simulink model "sea_tuning"  (R2014b)
settings: Solver=FixedStepDiscrete  StartTime=0.0  StopTime=inf  FixedStep=sample_time  RelTol=1e-3
undefined symbols (not defined in the file): A1_notch_f1, A2_notch_f1, B1_notch_f1, B2_notch_f1, back_left_triangle_period, back_left_triangle_wave_midpoint, back_left_triangle_wave_speed, back_right_triangle_period, back_right_triangle_wave_midpoint, back_right_triangle_wave_speed, boom_mount_angle, commanded_spring_torque, control_start_time, enable_left_step, enable_right_step, front_left_triangle_period, front_left_triangle_wave_midpoint, front_left_triangle_wave_speed, front_right_triangle_period, front_right_triangle_wave_midpoint, front_right_triangle_wave_speed, g, K_notch_f1, k_sea, kd_lateral, kd_sea_tuning, kd_swing_trajectory, kp_lateral, kp_sea_tuning, kp_swing_trajectory, l_seg, lateral_offset, lowest_commanded_spring_torque, m_leg_motor, max_sagittal_desired_swing_torque, max_sagittal_loaded_torque, max_sagittal_unloaded_torque, max_torque_lateral, maximum_lateral_angle, minimum_lateral_angle, sample_time, sea_coulomb_friction_direction_switch_sensitivity_tuning, sea_coulomb_friction_tuning, spring_torque_step_period
libraries: simulink x3
settings Model: xpc_rtwmakecfg_data=_xpcethercatlib_  BufferReuse=off  Creator=wmartin  LastModifiedBy=wmartin
settings SolverCC: EnableConcurrentExecution=on
settings DataIOCC: MaxDataPoints=1000000000  SaveFormat=StructureWithTime
settings OptimizationCC: BlockReduction=off  OptimizeBlockIOStorage=off  BufferReuse=off  GlobalBufferReuse=off  ExpressionFolding=off  ExpressionDepthLimit=2147483647  LocalBlockOutputs=off  SimCompilerOptimization=On
settings DebuggingCC: UnderspecifiedInitializationDetection=Classic  MergeDetectMultiDrivingBlocksExec=none  StateNameClashWarn=warning
settings HardwareCC: ProdIntDivRoundTo=Zero  ProdEndianess=LittleEndian  ProdLongLongMode=on  ProdHWDeviceType=Generic->32-bit x86 compatible
settings ModelReferenceCC: UpdateModelReferenceTargets=IfOutOfDate  EnableParallelModelReferenceBuilds=on
settings RTWCC: SystemTargetFile=slrt.tlc  TemplateMakefile=slrt_default_tmf  Description=Simulink Real-Time  RTWVerbose=off  ProcessScript=slrt_make_rtw_hook  RTWCompilerOptimization=On
settings CodeAppCC: MaxIdLength=256
settings SimulinkRealTimeCC: GeneratePreprocessorConditionals=Disable all  EnableShiftOperators=on  RL32LogBufSizeModifier=100000000

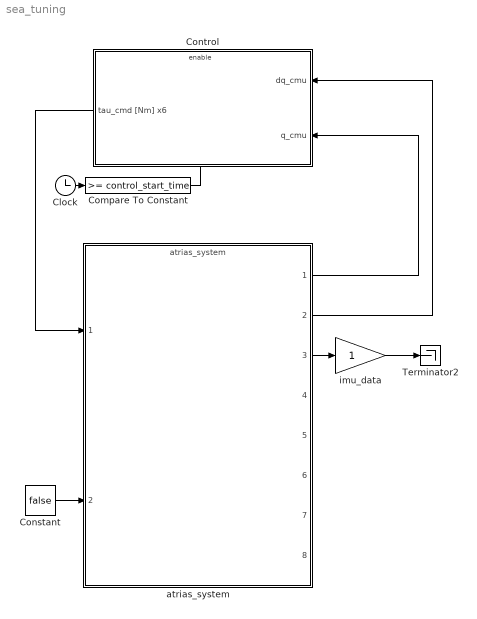
== system sea_tuning ==
  Clock : Clock
  Compare To Constant : simulink/Logic and Bit Operations/Compare To Constant  relop=>=  const=control_start_time  OutDataTypeStr=boolean
  Constant : Constant  Value=false
  Control : Subsystem
  Terminator2 : Terminator
  atrias_system : ModelReference  ModelNameDialog=atrias_system  SimulationMode=Normal  ModelReferenceVersion=1.2647  CopyOfModelName=atrias_system  DefaultDataLogging=on
  imu_data : Gain
  wires:
  Clock/1 -> Compare To Constant/1
  Compare To Constant/1 -> Control/Enable
  atrias_system/1 -> Control/2(q_cmu)
  atrias_system/2 -> Control/1(dq_cmu)
  Constant/1 -> atrias_system/2
  Control/1(tau_cmd [Nm] x6) -> atrias_system/1
  imu_data/1 -> Terminator2/1
  atrias_system/3 -> imu_data/1

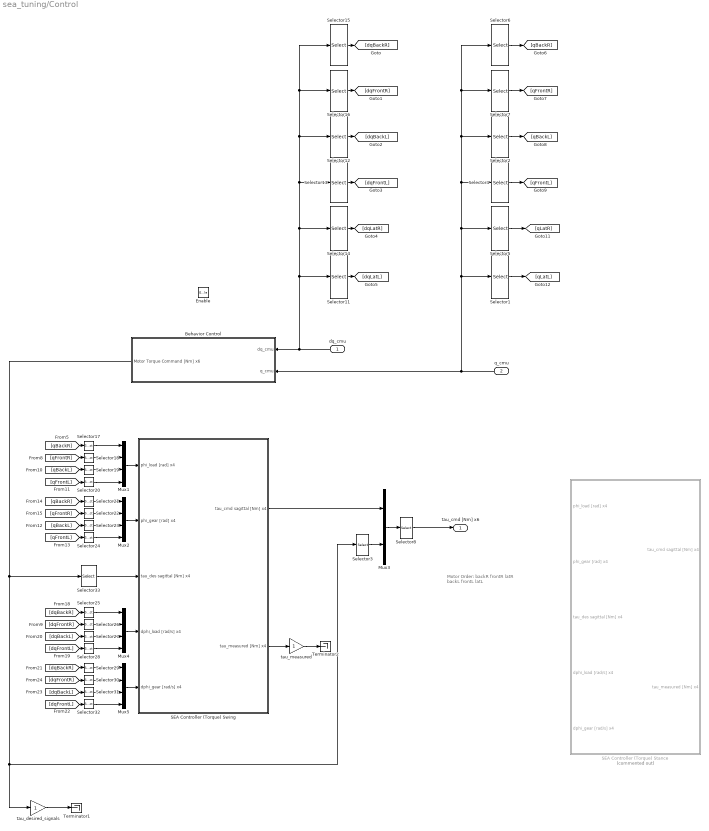
== system sea_tuning/Control ==
  note: Motor Order:
      |
      | backR
      | frontR
      | latR
      | backL
      | frontL
      | latL
  dq_cmu : Inport
  q_cmu : Inport  Port=2
  Enable : EnablePort  StatesWhenEnabling=reset
  Behavior Control : Subsystem
  Mux{1..2,4..5} (4 alike) : Mux
  Mux3 : Mux  Inputs=2
  SEA Controller (Torque) Stance : Subsystem  Commented=on
  SEA Controller (Torque) Swing : Subsystem
  Selector1 : Selector  InputPortWidth=13  Indices=[10]
  Selector11 : Selector  InputPortWidth=13  Indices=[10]
  Selector12 : Selector  InputPortWidth=13  Indices=[5 6]
  Selector13 : Selector  InputPortWidth=13  Indices=[7 8]
  Selector14 : Selector  InputPortWidth=13  Indices=[9]
  Selector15 : Selector  InputPortWidth=13  Indices=[1 2]
  Selector16 : Selector  InputPortWidth=13  Indices=[3 4]
  Selector{17..20,25..28} (8 alike) : Selector  InputPortWidth=2  Indices=[1]
  Selector2 : Selector  InputPortWidth=13  Indices=[5 6]
  Selector{21..24,29..32} (8 alike) : Selector  InputPortWidth=2  Indices=[2]
  Selector3 : Selector  InputPortWidth=6  Indices=[3 6]
  Selector33 : Selector  InputPortWidth=6  Indices=[1 2 4 5]
  Selector4 : Selector  InputPortWidth=13  Indices=[7 8]
  Selector5 : Selector  InputPortWidth=13  Indices=[9]
  Selector6 : Selector  InputPortWidth=13  Indices=[1 2]
  Selector7 : Selector  InputPortWidth=13  Indices=[3 4]
  Selector8 : Selector  InputPortWidth=6  Indices=[1 2 5 3 4 6]
  Terminator1 : Terminator
  Terminator2 : Terminator
  tau_desired_signals : Gain  Description=xPCTag(1)=tau_cmd_signal;
  tau_measured : Gain  Description=xPCTag(1)=tau_cmd_signal;
  tau_cmd [Nm] x6 : Outport  InitialOutput=[0 0 0 0 0 0]
  wires:
  SEA Controller (Torque) Swing/1(tau_cmd sagittal [Nm] x4) -> Mux3/1
  Behavior Control/1(Motor Torque Command [Nm] x6) -> tau_desired_signals/1, Selector3/1, Selector33/1
  Selector8/1 -> tau_cmd [Nm] x6/1
  tau_desired_signals/1 -> Terminator1/1
  Selector5/1 -> [qLatR]
  Selector1/1 -> [qLatL]
  Selector6/1 -> [qBackR]
  Selector7/1 -> [qFrontR]
  Selector2/1 -> [qBackL]
  Selector4/1 -> [qFrontL]
  q_cmu/1 -> Behavior Control/2(q_cmu), Selector2/1, Selector7/1, Selector6/1, Selector4/1, Selector5/1, Selector1/1
  dq_cmu/1 -> Selector15/1, Selector16/1, Selector12/1, Selector13/1, Selector14/1, Selector11/1, Behavior Control/1(dq_cmu)
  Selector14/1 -> [dqLatR]
  Selector11/1 -> [dqLatL]
  Selector15/1 -> [dqBackR]
  Selector16/1 -> [dqFrontR]
  Selector12/1 -> [dqBackL]
  Selector13/1 -> [dqFrontL]
  Mux1/1 -> SEA Controller (Torque) Swing/1(phi_load [rad] x4)
  [qBackR] -> Selector17/1
  Selector17/1 -> Mux1/1
  Selector19/1 -> Mux1/3
  Selector18/1 -> Mux1/2
  Selector20/1 -> Mux1/4
  [qFrontR] -> Selector18/1
  [qBackL] -> Selector19/1
  [qFrontL] -> Selector20/1
  Mux2/1 -> SEA Controller (Torque) Swing/2(phi_gear [rad] x4)
  [qBackR] -> Selector21/1
  Selector21/1 -> Mux2/1
  Selector23/1 -> Mux2/3
  Selector22/1 -> Mux2/2
  Selector24/1 -> Mux2/4
  [qFrontR] -> Selector22/1
  [qBackL] -> Selector23/1
  [qFrontL] -> Selector24/1
  Mux4/1 -> SEA Controller (Torque) Swing/4(dphi_load [rad/s] x4)
  [dqBackR] -> Selector25/1
  Selector25/1 -> Mux4/1
  Selector27/1 -> Mux4/3
  Selector26/1 -> Mux4/2
  Selector28/1 -> Mux4/4
  [dqFrontR] -> Selector26/1
  [dqBackL] -> Selector27/1
  [dqFrontL] -> Selector28/1
  Mux5/1 -> SEA Controller (Torque) Swing/5(dphi_gear [rad/s] x4)
  [dqBackR] -> Selector29/1
  Selector29/1 -> Mux5/1
  Selector31/1 -> Mux5/3
  Selector30/1 -> Mux5/2
  Selector32/1 -> Mux5/4
  [dqFrontR] -> Selector30/1
  [dqBackL] -> Selector31/1
  [dqFrontL] -> Selector32/1
  Selector33/1 -> SEA Controller (Torque) Swing/3(tau_des sagittal [Nm] x4)
  Selector3/1 -> Mux3/2
  Mux3/1 -> Selector8/1
  SEA Controller (Torque) Swing/2(tau_measured [Nm] x4) -> tau_measured/1
  tau_measured/1 -> Terminator2/1

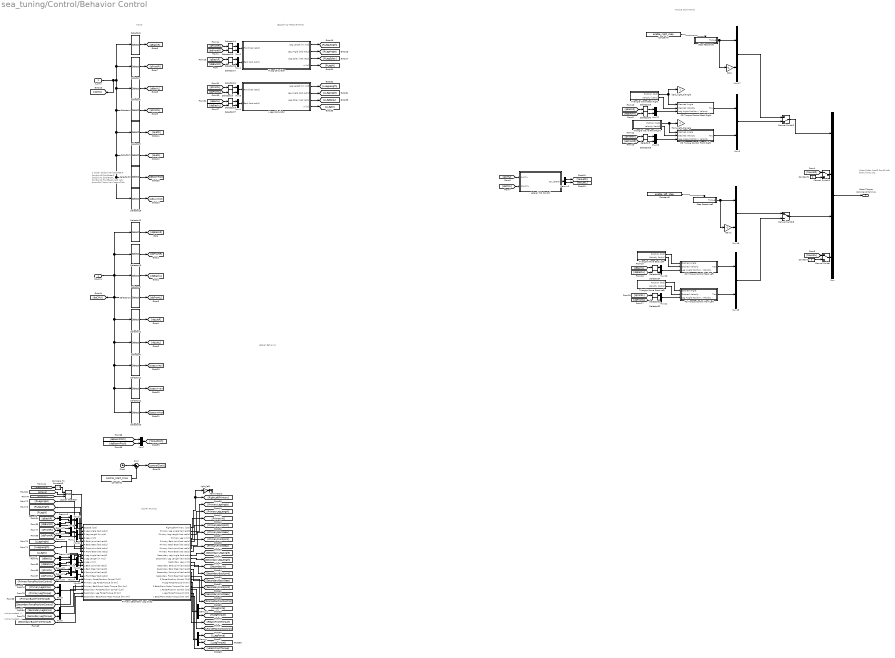
== system sea_tuning/Control/Behavior Control ==
  note: not connected -->
  note: Signal Routing
  note: Leg/Spring Measurements
  note: Lateral Behavior
  note: Torque Commands
  note: Inputs
  note: q Order:
      |
      | backJointR
      | backGearR
      | frontJointR
      | frontGearR
      |
      | backJointL
      | backGearL
      | frontJointL
      | frontGearL
      |
      | latR
      | latL
      |
      | boomRoll
      | boomYaw
      | boomPitch
  note: Motor Order:
      |
      | backR
      | frontR
      | latR
      | backL
      | frontL
      | latL
  note: not connected -->
  dq_cmu : Inport
  q_cmu : Inport  Port=2
  Clock : Clock
  Compare To Constant5 : simulink/Logic and Bit Operations/Compare To Constant  relop=>  const=2  OutDataTypeStr=boolean
  Constant : Constant  Value=0
  Constant1 : Constant  Value=0
  Constant2 : Constant  Value=control_start_time
  Constant4 : Constant  Value=enable_right_step
  Constant5 : Constant  Value=enable_left_step
  Demux{,1..10} (11 alike) : Demux  Outputs=2
  Gain : Gain  Gain=-1
  Gain1 : Gain  Gain=-1
  L Leg Calculator : Subsystem
  Lateral PID Control : Subsystem
  Logical Operator : Logic  Inputs=3  IconShape=distinctive  AllPortsSameDT=off  OutDataTypeStr=boolean
  Manual Switch : ManualSwitch
  Manual Switch1 : ManualSwitch
  Manual Switch2 : ManualSwitch  CurrentSetting=0
  Manual Switch3 : ManualSwitch
  Mux : Mux
  Mux{1..23} (23 alike) : Mux  Inputs=2
  PD Torque Control Back Left : Subsystem
  PD Torque Control Back Right : Subsystem
  PD Torque Control Front Left : Subsystem
  PD Torque Control Front Right : Subsystem
  Primary Secondary Leg Swap : Subsystem
  R Leg Calculator : Subsystem
  Selector1 : Selector  InputPortWidth=13  Indices=[10]
  Selector10 : Selector  InputPortWidth=13  Indices=[7 8]
  Selector11 : Selector  InputPortWidth=13  Indices=[9]
  Selector12 : Selector  InputPortWidth=13  Indices=[1 2]
  Selector13 : Selector  InputPortWidth=13  Indices=[3 4]
  Selector{3,14..17,24..34} (16 alike) : Selector  InputPortWidth=2  Indices=[1]
  Selector18 : Selector  InputPortWidth=13  Indices=[13]
  Selector2 : Selector  InputPortWidth=13  Indices=[5 6]
  Selector20 : Selector  InputPortWidth=13  Indices=[13]
  Selector21 : Selector  InputPortWidth=13  Indices=[11]
  Selector22 : Selector  InputPortWidth=13  Indices=[12]
  Selector23 : Selector  InputPortWidth=13  Indices=[11]
  Selector4 : Selector  InputPortWidth=13  Indices=[7 8]
  Selector5 : Selector  InputPortWidth=13  Indices=[9]
  Selector6 : Selector  InputPortWidth=13  Indices=[1 2]
  Selector7 : Selector  InputPortWidth=13  Indices=[3 4]
  Selector8 : Selector  InputPortWidth=13  Indices=[10]
  Selector9 : Selector  InputPortWidth=13  Indices=[5 6]
  Step Response : Subsystem
  Step Response2 : Subsystem
  Sum : Sum  Inputs=|+-
  Terminator2 : Terminator
  Triangle Wave Back Left : Subsystem
  Triangle Wave Back Right : Subsystem
  Triangle Wave Front Left : Subsystem
  Triangle Wave Front Right : Subsystem
  back_right_triangle : Gain
  front_right_triangle : Gain
  right_left : Gain
  Motor Torque Command [Nm] x6 : Outport  OutputWhenDisabled=reset  InitialOutput=[0 0 0 0 0 0]
  wires:
  [escape] -> Logical Operator/2
  Mux18/1 -> Manual Switch3/1
  Step Response2/1(Torque) -> Gain1/1, Mux18/1
  Step Response/1(Torque) -> Gain/1, Mux17/1
  Manual Switch/1 -> Mux/4
  Manual Switch1/1 -> Mux/2
  Mux17/1 -> Manual Switch2/1
  Primary Secondary Leg Swap/1(Right/Left Primary [1/0]) -> [RightLeftPrimary], right_left/1
  Logical Operator/1 -> Primary Secondary Leg Swap/1(escape [1/0])
  Primary Secondary Leg Swap/21(L Back/Front Motor Torque [Nm Nm]) -> [LBackFrontTorque]
  Primary Secondary Leg Swap/18(R Back/Front Motor Torque [Nm Nm]) -> [RBackFrontTorque]
  Primary Secondary Leg Swap/16(R Force/Position Control [1/0]) -> [RForcePositionControl]
  Primary Secondary Leg Swap/19(L Force/Position Control [1/0]) -> [LForcePositionControl]
  Primary Secondary Leg Swap/11(Secondary Leg w [m]) -> [SecondaryW]
  Primary Secondary Leg Swap/15(Secondary Front Gear [rad rad/s]) -> [SecondaryFrontGear]
  Primary Secondary Leg Swap/14(Secondary Front Joint [rad rad/s]) -> [SecondaryFrontJoint]
  Primary Secondary Leg Swap/13(Secondary Back Gear [rad rad/s]) -> [SecondaryBackGear]
  Primary Secondary Leg Swap/12(Secondary Back Joint [rad rad/s]) -> [SecondaryBackJoint]
  Primary Secondary Leg Swap/8(Primary Front Gear [rad rad/s]) -> [PrimaryFrontGear]
  Primary Secondary Leg Swap/7(Primary Front Joint [rad rad/s]) -> [PrimaryFrontJoint]
  Primary Secondary Leg Swap/6(Primary Back Gear [rad rad/s]) -> [PrimaryBackGear]
  Primary Secondary Leg Swap/5(Primary Back Joint [rad rad/s]) -> [PrimaryBackJoint]
  [SecondaryBackFrontTorque] -> Primary Secondary Leg Swap/21(Secondary Back/Front Motor Torque [Nm Nm])
  [PrimaryBackFrontTorque] -> Primary Secondary Leg Swap/18(Primary Back/Front Motor Torque [Nm Nm])
  [SecondaryForcePositionControl] -> Primary Secondary Leg Swap/19(Secondary Force/Position Control [1/0])
  [PrimaryForcePositionControl] -> Primary Secondary Leg Swap/16(Primary Force/Position Control [1/0])
  Demux9/2 -> Mux13/2
  Demux9/1 -> Mux16/2
  Demux10/2 -> Mux13/1
  Demux10/1 -> Mux16/1
  [qBackL] -> Demux10/1
  [dqBackL] -> Demux9/1
  Demux8/2 -> Mux15/2
  Demux8/1 -> Mux14/2
  Demux7/2 -> Mux15/1
  Demux7/1 -> Mux14/1
  Mux15/1 -> Primary Secondary Leg Swap/15(L Front Gear [rad rad/s])
  Mux14/1 -> Primary Secondary Leg Swap/14(L Front Joint [rad rad/s])
  Mux13/1 -> Primary Secondary Leg Swap/13(L Back Gear [rad rad/s])
  Mux16/1 -> Primary Secondary Leg Swap/12(L Back Joint [rad rad/s])
  [dqFrontL] -> Demux8/1
  [qFrontL] -> Demux7/1
  Demux5/2 -> Mux10/2
  Demux5/1 -> Mux9/2
  Demux6/2 -> Mux10/1
  Demux6/1 -> Mux9/1
  [qBackR] -> Demux6/1
  [dqBackR] -> Demux5/1
  Demux4/2 -> Mux12/2
  Demux4/1 -> Mux11/2
  Demux3/2 -> Mux12/1
  Demux3/1 -> Mux11/1
  Mux12/1 -> Primary Secondary Leg Swap/8(R Front Gear [rad rad/s])
  Mux11/1 -> Primary Secondary Leg Swap/7(R Front Joint [rad rad/s])
  Mux10/1 -> Primary Secondary Leg Swap/6(R Back Gear [rad rad/s])
  Mux9/1 -> Primary Secondary Leg Swap/5(R Back Joint [rad rad/s])
  [dqFrontR] -> Demux4/1
  [qFrontR] -> Demux3/1
  Demux1/2 -> [RLegTorque]
  Demux1/1 -> [RLegForce]
  Primary Secondary Leg Swap/17(R Leg Force/Torque [N Nm]) -> Demux1/1
  Demux/2 -> [LLegTorque]
  Demux/1 -> [LLegForce]
  Primary Secondary Leg Swap/20(L Leg Force/Torque [N Nm]) -> Demux/1
  Primary Secondary Leg Swap/9(Secondary Leg Angle [rad rad/s]) -> [SecondaryLegAngle]
  Primary Secondary Leg Swap/10(Secondary Leg Length [rad rad/s]) -> [SecondaryLegLength]
  [PrimaryLegForce] -> Mux8/1
  [PrimaryLegTorque] -> Mux8/2
  Mux8/1 -> Primary Secondary Leg Swap/17(Primary Leg Force/Torque [N Nm])
  Mux6/1 -> Primary Secondary Leg Swap/20(Secondary Leg Force/Torque [N Nm])
  [SecondaryLegTorque] -> Mux6/2
  [SecondaryLegForce] -> Mux6/1
  [LLegW] -> Primary Secondary Leg Swap/11(L Leg w [m])
  [LLegLength] -> Primary Secondary Leg Swap/10(L Leg Length [m m/s])
  [LLegAngle] -> Primary Secondary Leg Swap/9(L Leg Angle [rad rad/s])
  [RLegW] -> Primary Secondary Leg Swap/4(R Leg w [m])
  [RLegLength] -> Primary Secondary Leg Swap/3(R Leg Length [m m/s])
  [RLegAngle] -> Primary Secondary Leg Swap/2(R Leg Angle [rad rad/s])
  Primary Secondary Leg Swap/3(Primary Leg Length [rad rad/s]) -> [PrimaryLegLength]
  Primary Secondary Leg Swap/4(Primary Leg w [m]) -> [PrimaryW]
  Primary Secondary Leg Swap/2(Primary Leg Angle [rad rad/s]) -> [PrimaryLegAngle]
  Mux7/1 -> [TorsoPitch]
  [dqBoomPitch] -> Mux7/2
  [qBoomPitch] -> Mux7/1
  [hopping] -> Logical Operator/3
  right_left/1 -> Terminator2/1
  L Leg Calculator/4(w [m]) -> [LLegW]
  R Leg Calculator/4(w [m]) -> [RLegW]
  Selector26/1 -> Mux4/1
  Selector27/1 -> Mux4/2
  Selector25/1 -> Mux5/2
  Selector24/1 -> Mux5/1
  L Leg Calculator/3(Leg Splay [rad rad/s]) -> [LLegSplay]
  L Leg Calculator/2(Leg Angle [rad rad/s]) -> [LLegAngle]
  L Leg Calculator/1("Leg Length [m m/s] ") -> [LLegLength]
  Mux4/1 -> L Leg Calculator/2(Back [rad rad/s])
  Mux5/1 -> L Leg Calculator/1(Front [rad rad/s])
  [dqFrontL] -> Selector25/1
  [qFrontL] -> Selector24/1
  [dqBackL] -> Selector27/1
  [qBackL] -> Selector26/1
  Selector23/1 -> [qBoomRoll]
  Selector21/1 -> [dqBoomRoll]
  dq_cmu/1 -> Selector9/1, Selector13/1, Selector12/1, [dqCMU], Selector10/1, Selector11/1, Selector8/1, Selector21/1, Selector22/1, Selector20/1
  Selector22/1 -> [dqBoomYaw]
  Selector20/1 -> [dqBoomPitch]
  Selector18/1 -> [qBoomPitch]
  q_cmu/1 -> [qCMU], Selector1/1, Selector23/1, Selector18/1, Selector5/1, Selector4/1, Selector2/1, Selector7/1, Selector6/1
  Selector16/1 -> Mux1/1
  Selector17/1 -> Mux1/2
  Selector15/1 -> Mux2/2
  Selector14/1 -> Mux2/1
  [tauLatL] -> Manual Switch/1
  [tauLatR] -> Manual Switch1/1
  R Leg Calculator/3(Leg Splay [rad rad/s]) -> [RLegSplay]
  R Leg Calculator/2(Leg Angle [rad rad/s]) -> [RLegAngle]
  R Leg Calculator/1("Leg Length [m m/s] ") -> [RLegLength]
  Mux1/1 -> R Leg Calculator/2(Back [rad rad/s])
  Mux2/1 -> R Leg Calculator/1(Front [rad rad/s])
  [dqFrontR] -> Selector15/1
  [qFrontR] -> Selector14/1
  [dqBackR] -> Selector17/1
  [qBackR] -> Selector16/1
  Selector10/1 -> [dqFrontL]
  Selector9/1 -> [dqBackL]
  Selector13/1 -> [dqFrontR]
  Selector12/1 -> [dqBackR]
  Selector11/1 -> [dqLatR]
  Selector8/1 -> [dqLatL]
  Mux/1 -> Motor Torque Command [Nm] x6/1
  Constant/1 -> Manual Switch/2
  Constant1/1 -> Manual Switch1/2
  Clock/1 -> Sum/1
  Constant2/1 -> Sum/2
  Selector5/1 -> [qLatR]
  Selector1/1 -> [qLatL]
  Selector6/1 -> [qBackR]
  Selector7/1 -> [qFrontR]
  Selector2/1 -> [qBackL]
  Selector4/1 -> [qFrontL]
  Sum/1 -> [controlClock]
  [StepCount] -> Compare To Constant5/1
  Compare To Constant5/1 -> Logical Operator/1
  Constant4/1 -> Step Response/Enable
  Constant5/1 -> Step Response2/Enable
  Gain/1 -> Mux17/2
  Gain1/1 -> Mux18/2
  Manual Switch2/1 -> Mux/1
  Manual Switch3/1 -> Mux/3
  Mux3/1 -> Manual Switch2/2
  Mux19/1 -> Manual Switch3/2
  PD Torque Control Back Right/1(Tau) -> Mux3/1
  PD Torque Control Front Right/1(Tau) -> Mux3/2
  Selector33/1 -> Mux20/1
  Selector34/1 -> Mux20/2
  Selector31/1 -> Mux21/1
  Selector32/1 -> Mux21/2
  Triangle Wave Back Left/1(Position [rad]) -> PD Torque Control Back Left/1(Desired Angle)
  Triangle Wave Back Left/2(Velocity [rad/s]) -> PD Torque Control Back Left/2(Desired Velocity)
  Mux20/1 -> PD Torque Control Back Left/3(Leg Angle Position / Velocity)
  Mux21/1 -> PD Torque Control Front Left/3(Leg Angle Position / Velocity)
  Triangle Wave Front Left/2(Velocity [rad/s]) -> PD Torque Control Front Left/2(Desired Velocity)
  Triangle Wave Front Left/1(Position [rad]) -> PD Torque Control Front Left/1(Desired Angle)
  PD Torque Control Back Left/1(Tau) -> Mux19/1
  PD Torque Control Front Left/1(Tau) -> Mux19/2
  Selector29/1 -> Mux22/1
  Selector30/1 -> Mux22/2
  Mux22/1 -> PD Torque Control Back Right/3(Leg Angle Position / Velocity)
  Mux23/1 -> PD Torque Control Front Right/3(Leg Angle Position / Velocity)
  Triangle Wave Front Right/1(Position [rad]) -> front_right_triangle/1, PD Torque Control Front Right/1(Desired Angle)
  Triangle Wave Front Right/2(Velocity [rad/s]) -> PD Torque Control Front Right/2(Desired Velocity)
  Triangle Wave Back Right/1(Position [rad]) -> back_right_triangle/1, PD Torque Control Back Right/1(Desired Angle)
  Triangle Wave Back Right/2(Velocity [rad/s]) -> PD Torque Control Back Right/2(Desired Velocity)
  [dqFrontL] -> Selector32/1
  [qFrontL] -> Selector31/1
  [dqBackL] -> Selector34/1
  [qBackL] -> Selector33/1
  [dqFrontR] -> Selector28/1
  [qFrontR] -> Selector3/1
  [dqBackR] -> Selector30/1
  [qBackR] -> Selector29/1
  Selector28/1 -> Mux23/2
  Selector3/1 -> Mux23/1
  Lateral PID Control/1(tau_lateral) -> Demux2/1
  [dqCMU] -> Lateral PID Control/2(dq_cmu)
  [qCMU] -> Lateral PID Control/1(q_cmu)
  Demux2/1 -> [tauLatR]
  Demux2/2 -> [tauLatL]

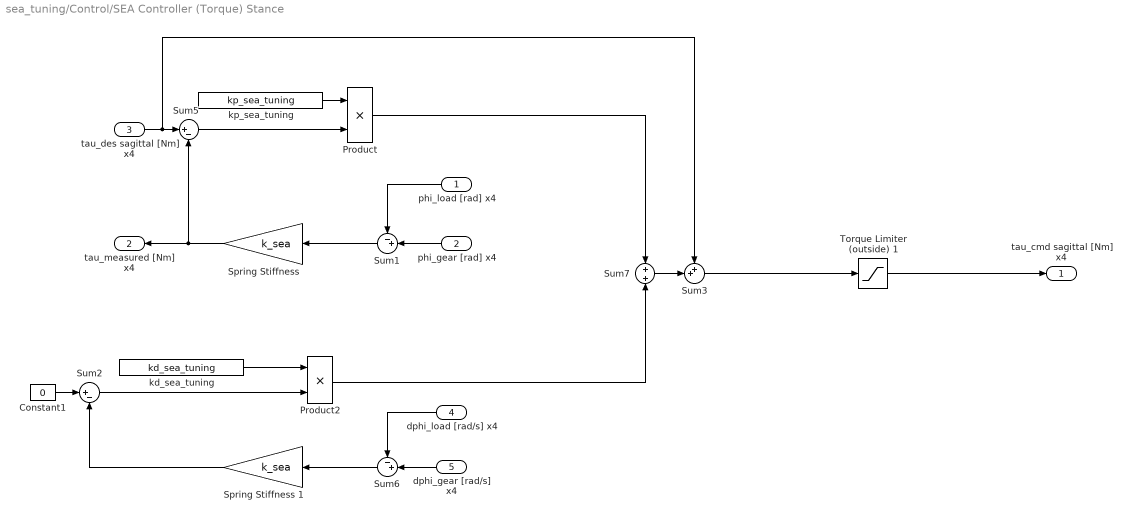
== system sea_tuning/Control/SEA Controller (Torque) Stance ==
  phi_load [rad] x4 : Inport
  phi_gear [rad] x4 : Inport  Port=2
  tau_des sagittal [Nm] x4 : Inport  Port=3
  dphi_load [rad/s] x4 : Inport  Port=4
  dphi_gear [rad/s] x4 : Inport  Port=5
  Constant1 : Constant  Value=0
  Product : Product  SampleTime=sample_time  RndMeth=Zero
  Product2 : Product  RndMeth=Zero
  Spring Stiffness : Gain  Gain=k_sea
  Spring Stiffness 1 : Gain  Gain=k_sea
  Sum1 : Sum  Inputs=-+|
  Sum2 : Sum  Inputs=|+-
  Sum3 : Sum  Inputs=++|
  Sum5 : Sum  Inputs=|+-
  Sum6 : Sum  Inputs=-+|
  Sum7 : Sum  Inputs=+|+
  Torque Limiter (outside) 1 : Saturate  UpperLimit=max_sagittal_loaded_torque  LowerLimit=-max_sagittal_loaded_torque
      settings: AttributesFormatString=Hi: %<UpperLimit>\nLo: %<LowerLimit>
  kd_sea_tuning : Constant  Value=kd_sea_tuning  SampleTime=sample_time
  kp_sea_tuning : Constant  Value=kp_sea_tuning  SampleTime=sample_time
  tau_cmd sagittal [Nm] x4 : Outport
  tau_measured [Nm] x4 : Outport  Port=2
  wires:
  Product2/1 -> Sum7/2
  kd_sea_tuning/1 -> Product2/1
  Sum2/1 -> Product2/2
  Sum5/1 -> Product/2
  dphi_gear [rad/s] x4/1 -> Sum6/2
  dphi_load [rad/s] x4/1 -> Sum6/1
  Spring Stiffness 1/1 -> Sum2/2
  Sum6/1 -> Spring Stiffness 1/1
  Constant1/1 -> Sum2/1
  tau_des sagittal [Nm] x4/1 -> Sum3/1, Sum5/1
  phi_gear [rad] x4/1 -> Sum1/2
  phi_load [rad] x4/1 -> Sum1/1
  Sum1/1 -> Spring Stiffness/1
  Spring Stiffness/1 -> Sum5/2, tau_measured [Nm] x4/1
  Sum3/1 -> Torque Limiter (outside) 1/1
  kp_sea_tuning/1 -> Product/1
  Product/1 -> Sum7/1
  Sum7/1 -> Sum3/2
  Torque Limiter (outside) 1/1 -> tau_cmd sagittal [Nm] x4/1

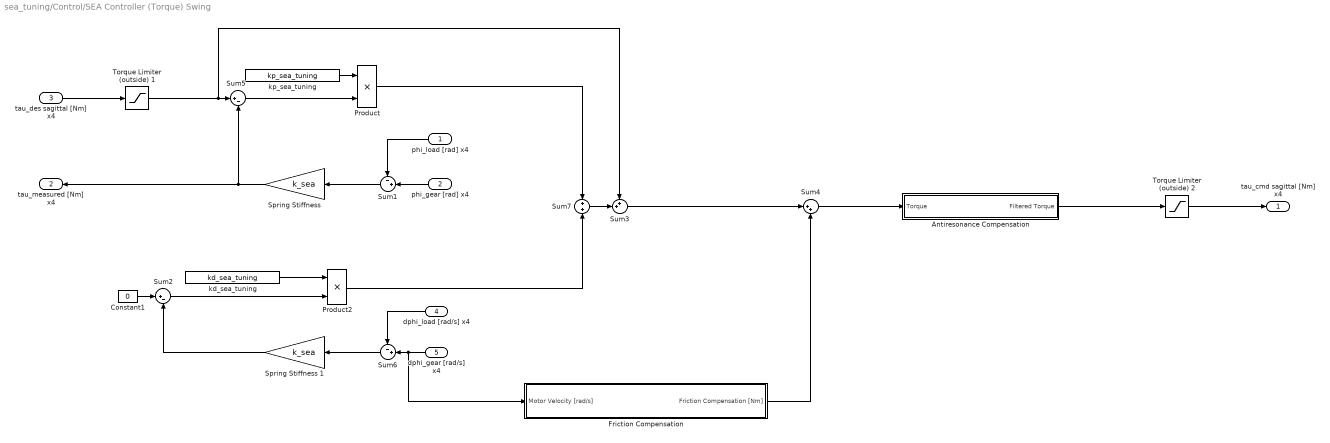
== system sea_tuning/Control/SEA Controller (Torque) Swing ==
  phi_load [rad] x4 : Inport
  phi_gear [rad] x4 : Inport  Port=2
  tau_des sagittal [Nm] x4 : Inport  Port=3
  dphi_load [rad/s] x4 : Inport  Port=4
  dphi_gear [rad/s] x4 : Inport  Port=5
  Antiresonance Compensation : Subsystem
  Constant1 : Constant  Value=0
  Friction Compensation : Subsystem
  Product : Product  SampleTime=sample_time  RndMeth=Zero
  Product2 : Product  RndMeth=Zero
  Spring Stiffness : Gain  Gain=k_sea
  Spring Stiffness 1 : Gain  Gain=k_sea
  Sum1 : Sum  Inputs=-+|
  Sum2 : Sum  Inputs=|+-
  Sum3 : Sum  Inputs=++|
  Sum4 : Sum  Inputs=|++
  Sum5 : Sum  Inputs=|+-
  Sum6 : Sum  Inputs=-+|
  Sum7 : Sum  Inputs=+|+
  Torque Limiter (outside) 1 : Saturate  UpperLimit=max_sagittal_desired_swing_torque  LowerLimit=-max_sagittal_desired_swing_torque
      settings: AttributesFormatString=Hi: %<UpperLimit>\nLo: %<LowerLimit>
  Torque Limiter (outside) 2 : Saturate  UpperLimit=max_sagittal_unloaded_torque  LowerLimit=-max_sagittal_unloaded_torque
      settings: AttributesFormatString=Hi: %<UpperLimit>\nLo: %<LowerLimit>
  kd_sea_tuning : Constant  Value=kd_sea_tuning  SampleTime=sample_time
  kp_sea_tuning : Constant  Value=kp_sea_tuning  SampleTime=sample_time
  tau_cmd sagittal [Nm] x4 : Outport
  tau_measured [Nm] x4 : Outport  Port=2
  wires:
  Product2/1 -> Sum7/2
  kd_sea_tuning/1 -> Product2/1
  Sum2/1 -> Product2/2
  Sum5/1 -> Product/2
  dphi_gear [rad/s] x4/1 -> Friction Compensation/1(Motor Velocity [rad/s]), Sum6/2
  dphi_load [rad/s] x4/1 -> Sum6/1
  Spring Stiffness 1/1 -> Sum2/2
  Sum6/1 -> Spring Stiffness 1/1
  Constant1/1 -> Sum2/1
  tau_des sagittal [Nm] x4/1 -> Torque Limiter (outside) 1/1
  phi_gear [rad] x4/1 -> Sum1/2
  phi_load [rad] x4/1 -> Sum1/1
  Sum1/1 -> Spring Stiffness/1
  Spring Stiffness/1 -> Sum5/2, tau_measured [Nm] x4/1
  Sum3/1 -> Sum4/1
  kp_sea_tuning/1 -> Product/1
  Product/1 -> Sum7/1
  Sum7/1 -> Sum3/2
  Torque Limiter (outside) 2/1 -> tau_cmd sagittal [Nm] x4/1
  Torque Limiter (outside) 1/1 -> Sum3/1, Sum5/1
  Antiresonance Compensation/1(Filtered Torque) -> Torque Limiter (outside) 2/1
  Sum4/1 -> Antiresonance Compensation/1(Torque)
  Friction Compensation/1(Friction Compensation [Nm]) -> Sum4/2

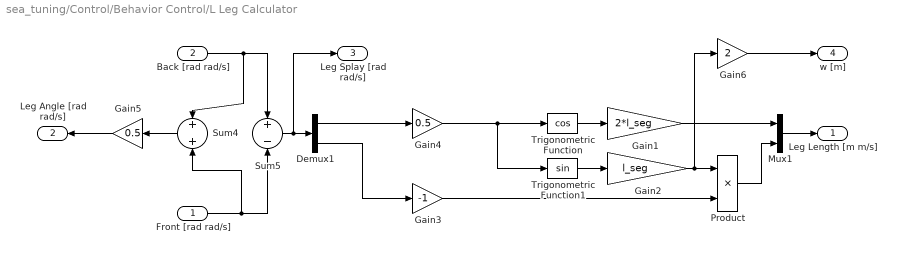
== system sea_tuning/Control/Behavior Control/L Leg Calculator ==
  Front [rad rad/s] : Inport
  Back [rad rad/s] : Inport  Port=2
  Demux1 : Demux  Outputs=2
  Gain1 : Gain  Gain=2*l_seg
  Gain2 : Gain  Gain=l_seg
  Gain3 : Gain  Gain=-1
  Gain4 : Gain  Gain=0.5
  Gain5 : Gain  Gain=0.5
  Gain6 : Gain  Gain=2
  Mux1 : Mux  Inputs=2
  Product : Product  RndMeth=Zero
  Sum4 : Sum  Inputs=+|+
  Sum5 : Sum  Inputs=+|-
  Trigonometric Function : Trigonometry  Operator=cos
  Trigonometric Function1 : Trigonometry
  "Leg Length [m m/s] " : Outport
  Leg Angle [rad rad/s] : Outport  Port=2
  Leg Splay [rad rad/s] : Outport  Port=3
  w [m] : Outport  Port=4
  wires:
  Gain6/1 -> w [m]/1
  Gain4/1 -> Trigonometric Function1/1, Trigonometric Function/1
  Trigonometric Function/1 -> Gain1/1
  Gain1/1 -> Mux1/1
  Trigonometric Function1/1 -> Gain2/1
  Product/1 -> Mux1/2
  Front [rad rad/s]/1 -> Sum5/2, Sum4/2
  Back [rad rad/s]/1 -> Sum4/1, Sum5/1
  Demux1/2 -> Gain3/1
  Gain3/1 -> Product/2
  Demux1/1 -> Gain4/1
  Gain2/1 -> Product/1, Gain6/1
  Sum5/1 -> Leg Splay [rad rad/s]/1, Demux1/1
  Mux1/1 -> "Leg Length [m m/s] "/1
  Sum4/1 -> Gain5/1
  Gain5/1 -> Leg Angle [rad rad/s]/1

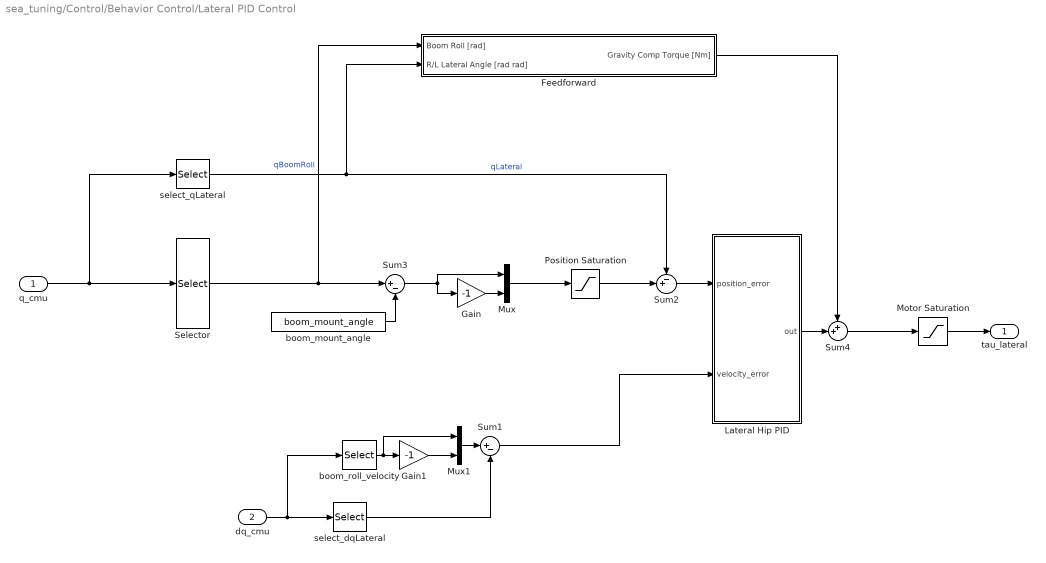
== system sea_tuning/Control/Behavior Control/Lateral PID Control ==
  q_cmu : Inport
  dq_cmu : Inport  Port=2
  Feedforward : Subsystem
  Gain : Gain  Gain=-1
  Gain1 : Gain  Gain=-1
  Lateral Hip PID : Subsystem
  Motor Saturation : Saturate  UpperLimit=max_torque_lateral  LowerLimit=-max_torque_lateral
      settings: AttributesFormatString=Top: %<UpperLimit>\nBottom: %<LowerLimit>
  Mux : Mux  Inputs=2
  Mux1 : Mux  Inputs=2
  Position Saturation : Saturate  UpperLimit=maximum_lateral_angle  LowerLimit=minimum_lateral_angle
      settings: AttributesFormatString=Top: %<UpperLimit>\nBottom: %<LowerLimit>
  Selector : Selector  InputPortWidth=13  Indices=[11]
  Sum1 : Sum  Inputs=|+-
  Sum2 : Sum  Inputs=-+|
  Sum3 : Sum  Inputs=|+-
  Sum4 : Sum  Inputs=++|
  boom_mount_angle : Constant  Value=boom_mount_angle
  boom_roll_velocity : Selector  InputPortWidth=13  Indices=[11]
  select_dqLateral : Selector  InputPortWidth=13  Indices=[9 10]
  select_qLateral : Selector  InputPortWidth=13  Indices=[9 10]
  tau_lateral : Outport
  wires:
  Selector/1 -> Sum3/1, Feedforward/1(Boom Roll [rad])  "qBoomRoll"
  q_cmu/1 -> Selector/1, select_qLateral/1
  boom_mount_angle/1 -> Sum3/2
  Feedforward/1(Gravity Comp Torque [Nm]) -> Sum4/1
  Gain1/1 -> Mux1/2
  Mux1/1 -> Sum1/1
  Sum3/1 -> Gain/1, Mux/1
  Motor Saturation/1 -> tau_lateral/1
  select_qLateral/1 -> Sum2/1, Feedforward/2(R/L Lateral Angle [rad rad])  "qLateral"
  Mux/1 -> Position Saturation/1
  Gain/1 -> Mux/2
  Sum1/1 -> Lateral Hip PID/2(velocity_error)
  boom_roll_velocity/1 -> Gain1/1, Mux1/1
  dq_cmu/1 -> boom_roll_velocity/1, select_dqLateral/1
  select_dqLateral/1 -> Sum1/2
  Sum2/1 -> Lateral Hip PID/1(position_error)
  Sum4/1 -> Motor Saturation/1
  Position Saturation/1 -> Sum2/2
  Lateral Hip PID/1(out) -> Sum4/2

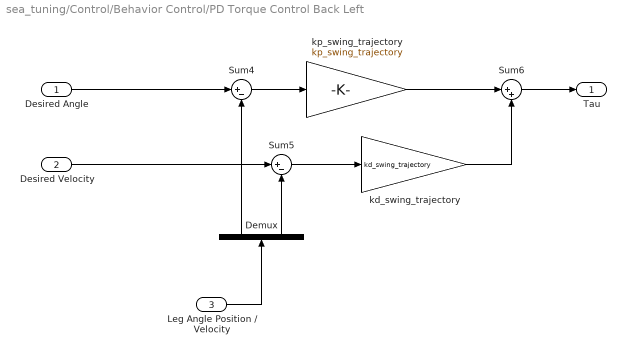
== system sea_tuning/Control/Behavior Control/PD Torque Control Back Left ==
  Desired Angle : Inport
  Desired Velocity : Inport  Port=2
  Leg Angle Position / Velocity : Inport  Port=3
  Demux : Demux  Outputs=2
  Sum4 : Sum  Inputs=|+-
  Sum5 : Sum  Inputs=|+-
  Sum6 : Sum  Inputs=|++
  kd_swing_trajectory : Gain  Gain=kd_swing_trajectory
  kp_swing_trajectory : Gain  Gain=kp_swing_trajectory
  Tau : Outport
  wires:
  Sum6/1 -> Tau/1
  Desired Angle/1 -> Sum4/1
  Demux/1 -> Sum4/2
  Leg Angle Position / Velocity/1 -> Demux/1
  Desired Velocity/1 -> Sum5/1
  Sum4/1 -> kp_swing_trajectory/1
  Sum5/1 -> kd_swing_trajectory/1
  kp_swing_trajectory/1 -> Sum6/1
  Demux/2 -> Sum5/2
  kd_swing_trajectory/1 -> Sum6/2

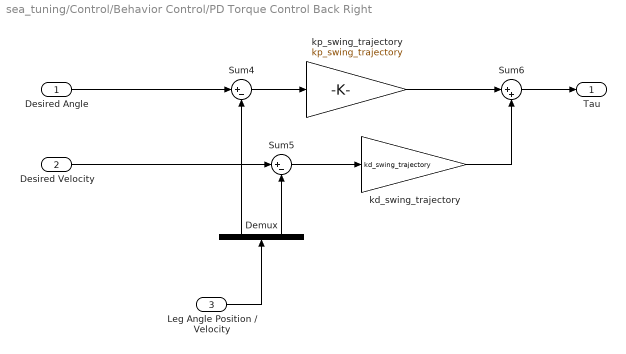
== system sea_tuning/Control/Behavior Control/PD Torque Control Back Right ==
  Desired Angle : Inport
  Desired Velocity : Inport  Port=2
  Leg Angle Position / Velocity : Inport  Port=3
  Demux : Demux  Outputs=2
  Sum4 : Sum  Inputs=|+-
  Sum5 : Sum  Inputs=|+-
  Sum6 : Sum  Inputs=|++
  kd_swing_trajectory : Gain  Gain=kd_swing_trajectory
  kp_swing_trajectory : Gain  Gain=kp_swing_trajectory
  Tau : Outport
  wires:
  kd_swing_trajectory/1 -> Sum6/2
  Demux/2 -> Sum5/2
  kp_swing_trajectory/1 -> Sum6/1
  Sum5/1 -> kd_swing_trajectory/1
  Sum4/1 -> kp_swing_trajectory/1
  Desired Velocity/1 -> Sum5/1
  Leg Angle Position / Velocity/1 -> Demux/1
  Demux/1 -> Sum4/2
  Desired Angle/1 -> Sum4/1
  Sum6/1 -> Tau/1

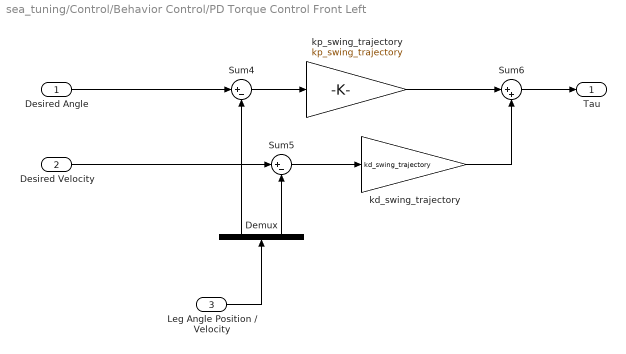
== system sea_tuning/Control/Behavior Control/PD Torque Control Front Left ==
  Desired Angle : Inport
  Desired Velocity : Inport  Port=2
  Leg Angle Position / Velocity : Inport  Port=3
  Demux : Demux  Outputs=2
  Sum4 : Sum  Inputs=|+-
  Sum5 : Sum  Inputs=|+-
  Sum6 : Sum  Inputs=|++
  kd_swing_trajectory : Gain  Gain=kd_swing_trajectory
  kp_swing_trajectory : Gain  Gain=kp_swing_trajectory
  Tau : Outport
  wires:
  kd_swing_trajectory/1 -> Sum6/2
  Demux/2 -> Sum5/2
  kp_swing_trajectory/1 -> Sum6/1
  Sum5/1 -> kd_swing_trajectory/1
  Sum4/1 -> kp_swing_trajectory/1
  Desired Velocity/1 -> Sum5/1
  Leg Angle Position / Velocity/1 -> Demux/1
  Demux/1 -> Sum4/2
  Desired Angle/1 -> Sum4/1
  Sum6/1 -> Tau/1

== system sea_tuning/Control/Behavior Control/PD Torque Control Front Right ==
  Desired Angle : Inport
  Desired Velocity : Inport  Port=2
  Leg Angle Position / Velocity : Inport  Port=3
  Demux : Demux  Outputs=2
  Sum4 : Sum  Inputs=|+-
  Sum5 : Sum  Inputs=|+-
  Sum6 : Sum  Inputs=|++
  kd_swing_trajectory : Gain  Gain=kd_swing_trajectory
  kp_swing_trajectory : Gain  Gain=kp_swing_trajectory
  Tau : Outport
  wires:
  Sum6/1 -> Tau/1
  Desired Angle/1 -> Sum4/1
  Demux/1 -> Sum4/2
  Leg Angle Position / Velocity/1 -> Demux/1
  Desired Velocity/1 -> Sum5/1
  Sum4/1 -> kp_swing_trajectory/1
  Sum5/1 -> kd_swing_trajectory/1
  kp_swing_trajectory/1 -> Sum6/1
  Demux/2 -> Sum5/2
  kd_swing_trajectory/1 -> Sum6/2

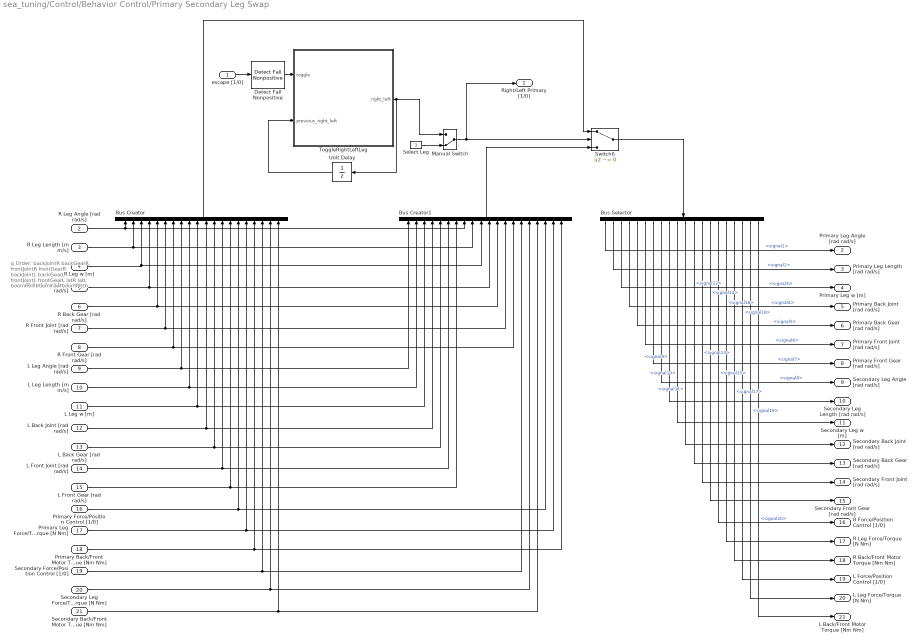
== system sea_tuning/Control/Behavior Control/Primary Secondary Leg Swap ==
  note: q Order:
      |
      | backJointR
      | backGearR
      | frontJointR
      | frontGearR
      |
      | backJointL
      | backGearL
      | frontJointL
      | frontGearL
      |
      | latR
      | latL
      |
      | boomRoll
      | boomYaw
      | boomPitch
  escape [1/0] : Inport
  R Leg Angle [rad rad/s] : Inport  Port=2
  R Leg Length [m m/s] : Inport  Port=3
  R Leg w [m] : Inport  Port=4
  R Back Joint [rad rad/s] : Inport  Port=5
  R Back Gear [rad rad/s] : Inport  Port=6
  R Front Joint [rad rad/s] : Inport  Port=7
  R Front Gear [rad rad/s] : Inport  Port=8
  L Leg Angle [rad rad/s] : Inport  Port=9
  L Leg Length [m m/s] : Inport  Port=10
  L Leg w [m] : Inport  Port=11
  L Back Joint [rad rad/s] : Inport  Port=12
  L Back Gear [rad rad/s] : Inport  Port=13
  L Front Joint [rad rad/s] : Inport  Port=14
  L Front Gear [rad rad/s] : Inport  Port=15
  Primary Force/Position Control [1/0] : Inport  Port=16
  Primary Leg Force/Torque [N Nm] : Inport  Port=17
  Primary Back/Front Motor Torque [Nm Nm] : Inport  Port=18
  Secondary Force/Position Control [1/0] : Inport  Port=19
  Secondary Leg Force/Torque [N Nm] : Inport  Port=20
  Secondary Back/Front Motor Torque [Nm Nm] : Inport  Port=21
  Bus Creator : BusCreator  Inputs=20
  Bus Creator1 : BusCreator  Inputs=20
  Bus Selector : BusSelector  OutputSignals=signal1,signal2,signal3,signal4,signal5,signal6,signal7,signal8,signal9,signal10,signal11,signal12,signal13,signal14,signal15,signal16,signal17,signal18,signal19,signal20
  Detect Fall Nonpositive : simulink/Logic and Bit Operations/Detect Fall Nonpositive  vinit=0  InputProcessing=Inherited  OutDataTypeStr=boolean
  Manual Switch : ManualSwitch  CurrentSetting=0
  Select Leg : Constant  OutDataTypeStr=boolean
  Switch6 : Switch  Criteria=u2 ~= 0  OutDataTypeStr=Inherit: Inherit via back propagation  ZeroCross=off
  ToggleRightLeftLeg : MATLAB Function  TreatAsAtomicUnit=on
      settings: MinAlgLoopOccurrences=on
  Unit Delay : UnitDelay  SampleTime=sample_time
  Right/Left Primary [1/0] : Outport
  Primary Leg Angle [rad rad/s] : Outport  Port=2
  Primary Leg Length [rad rad/s] : Outport  Port=3
  Primary Leg w [m] : Outport  Port=4
  Primary Back Joint [rad rad/s] : Outport  Port=5
  Primary Back Gear [rad rad/s] : Outport  Port=6
  Primary Front Joint [rad rad/s] : Outport  Port=7
  Primary Front Gear [rad rad/s] : Outport  Port=8
  Secondary Leg Angle [rad rad/s] : Outport  Port=9
  Secondary Leg Length [rad rad/s] : Outport  Port=10
  Secondary Leg w [m] : Outport  Port=11
  Secondary Back Joint [rad rad/s] : Outport  Port=12
  Secondary Back Gear [rad rad/s] : Outport  Port=13
  Secondary Front Joint [rad rad/s] : Outport  Port=14
  Secondary Front Gear [rad rad/s] : Outport  Port=15
  R Force/Position Control [1/0] : Outport  Port=16
  R Leg Force/Torque [N Nm] : Outport  Port=17
  R Back/Front Motor Torque [Nm Nm] : Outport  Port=18
  L Force/Position Control [1/0] : Outport  Port=19
  L Leg Force/Torque [N Nm] : Outport  Port=20
  L Back/Front Motor Torque [Nm Nm] : Outport  Port=21
  wires:
  Unit Delay/1 -> ToggleRightLeftLeg/2(previous_right_left)
  Detect Fall Nonpositive/1 -> ToggleRightLeftLeg/1(toggle)
  escape [1/0]/1 -> Detect Fall Nonpositive/1
  ToggleRightLeftLeg/1(right_left) -> Unit Delay/1, Manual Switch/1
  Manual Switch/1 -> Right/Left Primary [1/0]/1, Switch6/2
  Select Leg/1 -> Manual Switch/2
  R Leg w [m]/1 -> Bus Creator1/10, Bus Creator/3
  R Leg Angle [rad rad/s]/1 -> Bus Creator1/8, Bus Creator/1
  R Leg Length [m m/s]/1 -> Bus Creator1/9, Bus Creator/2
  Bus Creator/1 -> Switch6/1
  Bus Creator1/1 -> Switch6/3
  R Back Joint [rad rad/s]/1 -> Bus Creator1/11, Bus Creator/4
  R Back Gear [rad rad/s]/1 -> Bus Creator1/12, Bus Creator/5
  R Front Joint [rad rad/s]/1 -> Bus Creator1/13, Bus Creator/6
  R Front Gear [rad rad/s]/1 -> Bus Creator1/14, Bus Creator/7
  L Leg Angle [rad rad/s]/1 -> Bus Creator1/1, Bus Creator/8
  L Leg Length [m m/s]/1 -> Bus Creator1/2, Bus Creator/9
  L Leg w [m]/1 -> Bus Creator1/3, Bus Creator/10
  L Back Joint [rad rad/s]/1 -> Bus Creator1/4, Bus Creator/11
  L Back Gear [rad rad/s]/1 -> Bus Creator1/5, Bus Creator/12
  L Front Joint [rad rad/s]/1 -> Bus Creator/13, Bus Creator1/6
  L Front Gear [rad rad/s]/1 -> Bus Creator1/7, Bus Creator/14
  Primary Force/Position Control [1/0]/1 -> Bus Creator1/18, Bus Creator/15
  Primary Leg Force/Torque [N Nm]/1 -> Bus Creator1/19, Bus Creator/16
  Primary Back/Front Motor Torque [Nm Nm]/1 -> Bus Creator1/20, Bus Creator/17
  Secondary Force/Position Control [1/0]/1 -> Bus Creator1/15, Bus Creator/18
  Secondary Leg Force/Torque [N Nm]/1 -> Bus Creator1/16, Bus Creator/19
  Secondary Back/Front Motor Torque [Nm Nm]/1 -> Bus Creator1/17, Bus Creator/20
  Switch6/1 -> Bus Selector/1
  Bus Selector/1 -> Primary Leg Angle [rad rad/s]/1  "<signal1>"
  Bus Selector/2 -> Primary Leg Length [rad rad/s]/1  "<signal2>"
  Bus Selector/3 -> Primary Leg w [m]/1  "<signal3>"
  Bus Selector/4 -> Primary Back Joint [rad rad/s]/1  "<signal4>"
  Bus Selector/5 -> Primary Back Gear [rad rad/s]/1  "<signal5>"
  Bus Selector/6 -> Primary Front Joint [rad rad/s]/1  "<signal6>"
  Bus Selector/7 -> Primary Front Gear [rad rad/s]/1  "<signal7>"
  Bus Selector/8 -> Secondary Leg Angle [rad rad/s]/1  "<signal8>"
  Bus Selector/9 -> Secondary Leg Length [rad rad/s]/1  "<signal9>"
  Bus Selector/10 -> Secondary Leg w [m]/1  "<signal10>"
  Bus Selector/11 -> Secondary Back Joint [rad rad/s]/1  "<signal11>"
  Bus Selector/12 -> Secondary Back Gear [rad rad/s]/1  "<signal12>"
  Bus Selector/13 -> Secondary Front Joint [rad rad/s]/1  "<signal13>"
  Bus Selector/14 -> Secondary Front Gear [rad rad/s]/1  "<signal14>"
  Bus Selector/15 -> R Force/Position Control [1/0]/1  "<signal15>"
  Bus Selector/16 -> R Leg Force/Torque [N Nm]/1  "<signal16>"
  Bus Selector/17 -> R Back/Front Motor Torque [Nm Nm]/1  "<signal17>"
  Bus Selector/18 -> L Force/Position Control [1/0]/1  "<signal18>"
  Bus Selector/19 -> L Leg Force/Torque [N Nm]/1  "<signal19>"
  Bus Selector/20 -> L Back/Front Motor Torque [Nm Nm]/1  "<signal20>"

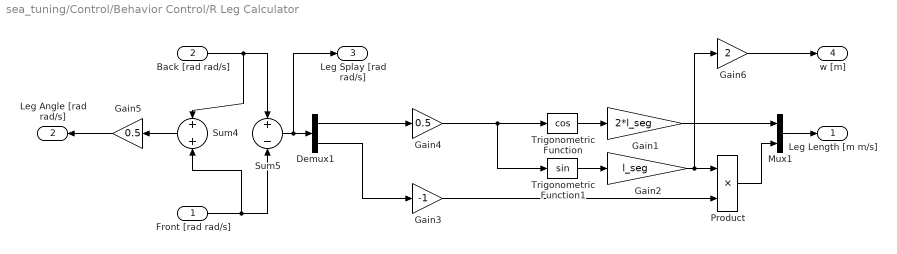
== system sea_tuning/Control/Behavior Control/R Leg Calculator ==
  Front [rad rad/s] : Inport
  Back [rad rad/s] : Inport  Port=2
  Demux1 : Demux  Outputs=2
  Gain1 : Gain  Gain=2*l_seg
  Gain2 : Gain  Gain=l_seg
  Gain3 : Gain  Gain=-1
  Gain4 : Gain  Gain=0.5
  Gain5 : Gain  Gain=0.5
  Gain6 : Gain  Gain=2
  Mux1 : Mux  Inputs=2
  Product : Product  RndMeth=Zero
  Sum4 : Sum  Inputs=+|+
  Sum5 : Sum  Inputs=+|-
  Trigonometric Function : Trigonometry  Operator=cos
  Trigonometric Function1 : Trigonometry
  "Leg Length [m m/s] " : Outport
  Leg Angle [rad rad/s] : Outport  Port=2
  Leg Splay [rad rad/s] : Outport  Port=3
  w [m] : Outport  Port=4
  wires:
  Gain5/1 -> Leg Angle [rad rad/s]/1
  Sum4/1 -> Gain5/1
  Mux1/1 -> "Leg Length [m m/s] "/1
  Sum5/1 -> Demux1/1, Leg Splay [rad rad/s]/1
  Gain2/1 -> Gain6/1, Product/1
  Demux1/1 -> Gain4/1
  Gain3/1 -> Product/2
  Demux1/2 -> Gain3/1
  Back [rad rad/s]/1 -> Sum5/1, Sum4/1
  Front [rad rad/s]/1 -> Sum4/2, Sum5/2
  Product/1 -> Mux1/2
  Trigonometric Function1/1 -> Gain2/1
  Gain1/1 -> Mux1/1
  Trigonometric Function/1 -> Gain1/1
  Gain4/1 -> Trigonometric Function/1, Trigonometric Function1/1
  Gain6/1 -> w [m]/1

== system sea_tuning/Control/Behavior Control/Step Response ==
  Enable : EnablePort  StatesWhenEnabling=reset  ShowOutputPort=on
  Constant : Constant  Value=lowest_commanded_spring_torque
  Pulse Generator : DiscretePulseGenerator  PulseType=Time based  TimeSource=Use external signal  Amplitude=commanded_spring_torque  Period=spring_torque_step_period  PulseWidth=50
  Sum : Sum  Inputs=|++
  Timer : Subsystem
  Torque : Outport  OutputWhenDisabled=reset  InitialOutput=[0]
  wires:
  Timer/1(timer [s]) -> Pulse Generator/1
  Enable/1 -> Timer/Enable
  Pulse Generator/1 -> Sum/1
  Sum/1 -> Torque/1
  Constant/1 -> Sum/2

== system sea_tuning/Control/Behavior Control/Step Response2 ==
  Enable : EnablePort  StatesWhenEnabling=reset  ShowOutputPort=on
  Constant : Constant  Value=lowest_commanded_spring_torque
  Pulse Generator : DiscretePulseGenerator  PulseType=Time based  TimeSource=Use external signal  Amplitude=commanded_spring_torque  Period=spring_torque_step_period  PulseWidth=50
  Sum : Sum  Inputs=|++
  Timer : Subsystem
  Torque : Outport  OutputWhenDisabled=reset  InitialOutput=[0]
  wires:
  Constant/1 -> Sum/2
  Sum/1 -> Torque/1
  Pulse Generator/1 -> Sum/1
  Enable/1 -> Timer/Enable
  Timer/1(timer [s]) -> Pulse Generator/1

== system sea_tuning/Control/Behavior Control/Triangle Wave Back Left ==
  Constant1 : Constant  Value=0
  Constant5 : Constant  Value=-1
  Constant6 : Constant
  Direction : DiscretePulseGenerator  PulseType=Time based  Period=back_left_triangle_period  PulseWidth=50  PhaseDelay=back_left_triangle_period/4
  Manual Switch : ManualSwitch
  Speed : Gain  Gain=back_left_triangle_wave_speed
  Switch : Switch  Criteria=u2 ~= 0
  Triangle Wave : DiscreteIntegrator  InitialCondition=back_left_triangle_wave_midpoint  InitialConditionSetting=State (most efficient)  SampleTime=sample_time
  Position [rad] : Outport
  Velocity [rad/s] : Outport  Port=2
  wires:
  Speed/1 -> Manual Switch/1
  Constant1/1 -> Manual Switch/2
  Constant6/1 -> Switch/1
  Switch/1 -> Speed/1
  Direction/1 -> Switch/2
  Manual Switch/1 -> Triangle Wave/1, Velocity [rad/s]/1
  Constant5/1 -> Switch/3
  Triangle Wave/1 -> Position [rad]/1

== system sea_tuning/Control/Behavior Control/Triangle Wave Back Right ==
  Constant1 : Constant  Value=0
  Constant5 : Constant  Value=-1
  Constant6 : Constant
  Direction : DiscretePulseGenerator  PulseType=Time based  Period=back_right_triangle_period  PulseWidth=50  PhaseDelay=back_right_triangle_period/4
  Manual Switch : ManualSwitch
  Speed : Gain  Gain=back_right_triangle_wave_speed
  Switch : Switch  Criteria=u2 ~= 0
  Triangle Wave : DiscreteIntegrator  InitialCondition=back_right_triangle_wave_midpoint  InitialConditionSetting=State (most efficient)  SampleTime=sample_time
  Position [rad] : Outport
  Velocity [rad/s] : Outport  Port=2
  wires:
  Constant1/1 -> Manual Switch/2
  Speed/1 -> Manual Switch/1
  Triangle Wave/1 -> Position [rad]/1
  Constant5/1 -> Switch/3
  Manual Switch/1 -> Triangle Wave/1, Velocity [rad/s]/1
  Direction/1 -> Switch/2
  Switch/1 -> Speed/1
  Constant6/1 -> Switch/1

== system sea_tuning/Control/Behavior Control/Triangle Wave Front Left ==
  Constant1 : Constant  Value=0
  Constant5 : Constant  Value=-1
  Constant6 : Constant
  Direction : DiscretePulseGenerator  PulseType=Time based  Period=front_left_triangle_period  PulseWidth=50  PhaseDelay=front_left_triangle_period/4
  Manual Switch : ManualSwitch
  Speed : Gain  Gain=front_left_triangle_wave_speed
  Switch : Switch  Criteria=u2 ~= 0
  Triangle Wave : DiscreteIntegrator  InitialCondition=front_left_triangle_wave_midpoint  InitialConditionSetting=State (most efficient)  SampleTime=sample_time
  Position [rad] : Outport
  Velocity [rad/s] : Outport  Port=2
  wires:
  Speed/1 -> Manual Switch/1
  Constant1/1 -> Manual Switch/2
  Triangle Wave/1 -> Position [rad]/1
  Constant5/1 -> Switch/3
  Manual Switch/1 -> Triangle Wave/1, Velocity [rad/s]/1
  Direction/1 -> Switch/2
  Switch/1 -> Speed/1
  Constant6/1 -> Switch/1

== system sea_tuning/Control/Behavior Control/Triangle Wave Front Right ==
  Constant1 : Constant  Value=0
  Constant5 : Constant  Value=-1
  Constant6 : Constant
  Direction : DiscretePulseGenerator  PulseType=Time based  Period=front_right_triangle_period  PulseWidth=50  PhaseDelay=front_right_triangle_period/4
  Manual Switch : ManualSwitch
  Speed : Gain  Gain=front_right_triangle_wave_speed
  Switch : Switch  Criteria=u2 ~= 0
  Triangle Wave : DiscreteIntegrator  InitialCondition=front_right_triangle_wave_midpoint  InitialConditionSetting=State (most efficient)  SampleTime=sample_time
  Position [rad] : Outport
  Velocity [rad/s] : Outport  Port=2
  wires:
  Speed/1 -> Manual Switch/1
  Constant1/1 -> Manual Switch/2
  Constant6/1 -> Switch/1
  Switch/1 -> Speed/1
  Direction/1 -> Switch/2
  Manual Switch/1 -> Triangle Wave/1, Velocity [rad/s]/1
  Constant5/1 -> Switch/3
  Triangle Wave/1 -> Position [rad]/1

== system sea_tuning/Control/SEA Controller (Torque) Swing/Antiresonance Compensation ==
  Torque : Inport
  Notch Filter (Flight) : DiscreteTransferFcn  Numerator=[K_notch_f1 K_notch_f1*A1_notch_f1 K_notch_f1*A2_notch_f1]  Denominator=[1 B1_notch_f1 B2_notch_f1]  SampleTime=sample_time
  Filtered Torque : Outport
  wires:
  Torque/1 -> Notch Filter (Flight)/1
  Notch Filter (Flight)/1 -> Filtered Torque/1

== system sea_tuning/Control/SEA Controller (Torque) Swing/Friction Compensation ==
  Motor Velocity [rad/s] : Inport
  Gain2 : Gain  Gain=sea_coulomb_friction_direction_switch_sensitivity_tuning
  KdGain2 : Gain  Description=xPCTag(1)=kd_sea_torque;  Gain=sea_coulomb_friction_tuning
  Trigonometric Function : Trigonometry  Operator=tanh
  Friction Compensation [Nm] : Outport
  wires:
  KdGain2/1 -> Friction Compensation [Nm]/1
  Motor Velocity [rad/s]/1 -> Gain2/1
  Gain2/1 -> Trigonometric Function/1
  Trigonometric Function/1 -> KdGain2/1

== system sea_tuning/Control/Behavior Control/Lateral PID Control/Feedforward ==
  Boom Roll [rad] : Inport
  R/L Lateral Angle [rad rad] : Inport  Port=2
  -mgd : Gain  Gain=m_leg_motor*g*lateral_offset
  Gain2 : Gain  Gain=[-1 1]
  Sum1 : Sum  Inputs=++|
  Sum3 : Sum  Inputs=++|
  boom_mount_angle : Constant  Value=boom_mount_angle
  sin : Trigonometry  Operator=cos
  Gravity Comp Torque [Nm] : Outport
  wires:
  Sum3/1 -> sin/1
  Gain2/1 -> Sum3/1
  Sum1/1 -> Gain2/1
  Boom Roll [rad]/1 -> Sum1/2
  R/L Lateral Angle [rad rad]/1 -> Sum3/2
  sin/1 -> -mgd/1
  -mgd/1 -> Gravity Comp Torque [Nm]/1
  boom_mount_angle/1 -> Sum1/1

== system sea_tuning/Control/Behavior Control/Lateral PID Control/Lateral Hip PID ==
  position_error : Inport
  velocity_error : Inport  Port=2
  Sum : Sum  Inputs=++|
  kd_lateral : Gain  Description=xPCTag(1)=kd_lateral;  Gain=kd_lateral
  kp_lateral : Gain  Description=xPCTag(1)=kp_lateral;  Gain=kp_lateral
  out : Outport
  wires:
  kd_lateral/1 -> Sum/1
  Sum/1 -> out/1
  position_error/1 -> kp_lateral/1
  kp_lateral/1 -> Sum/2
  velocity_error/1 -> kd_lateral/1

== system sea_tuning/Control/Behavior Control/Step Response/Timer ==
  Enable : EnablePort  StatesWhenEnabling=reset  ShowOutputPort=on
  Constant : Constant
  Discrete-Time Integrator : DiscreteIntegrator  IntegratorMethod=Accumulation: Forward Euler  gainval=sample_time  ExternalReset=rising  SampleTime=sample_time
  timer [s] : Outport  InitialOutput=[0]
  wires:
  Discrete-Time Integrator/1 -> timer [s]/1
  Enable/1 -> Discrete-Time Integrator/2
  Constant/1 -> Discrete-Time Integrator/1

== system sea_tuning/Control/Behavior Control/Step Response2/Timer ==
  Enable : EnablePort  StatesWhenEnabling=reset  ShowOutputPort=on
  Constant : Constant
  Discrete-Time Integrator : DiscreteIntegrator  IntegratorMethod=Accumulation: Forward Euler  gainval=sample_time  ExternalReset=rising  SampleTime=sample_time
  timer [s] : Outport  InitialOutput=[0]
  wires:
  Constant/1 -> Discrete-Time Integrator/1
  Enable/1 -> Discrete-Time Integrator/2
  Discrete-Time Integrator/1 -> timer [s]/1

== matlab function sea_tuning/Control/Behavior Control/Primary Secondary Leg Swap/ToggleRightLeftLeg ==
  data: toggle input boolean; right_left output double; previous_right_left input double
function right_left = ToggleRightLeftLeg(toggle, previous_right_left)
    
    if toggle
        right_left = -previous_right_left + 1;
    else
        right_left = previous_right_left;
    end

end
